simulink model "MovimientoTraslacionalSimulink2"  (R2023a)
settings: Solver=VariableStepAuto  StartTime=0.0  StopTime=10.0  RelTol=1e-3
values from neighbouring files (symbols this model uses):
  b1 = 1000    [MovTrasODE45.m]    (also in MovimientoTraslacionalSimulink.m)
  k1 = 16182    [MovTrasODE45.m]    (also in MovimientoTraslacionalSimulink.m)
  k2 = 19000    [MovTrasODE45.m]    (also in MovimientoTraslacionalSimulink.m)
  m1 = 290    [MovTrasODE45.m]    (also in MovimientoTraslacionalSimulink.m)
  m2 = 59    [MovTrasODE45.m]    (also in MovimientoTraslacionalSimulink.m)
settings Model: Creator=josel
settings OptimizationCC: ReuseModelBlockBuffer=off

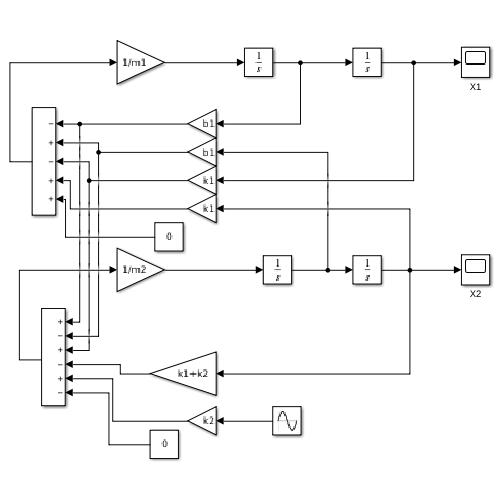
[thumbnail: Simulink's stored preview of the top-level diagram]
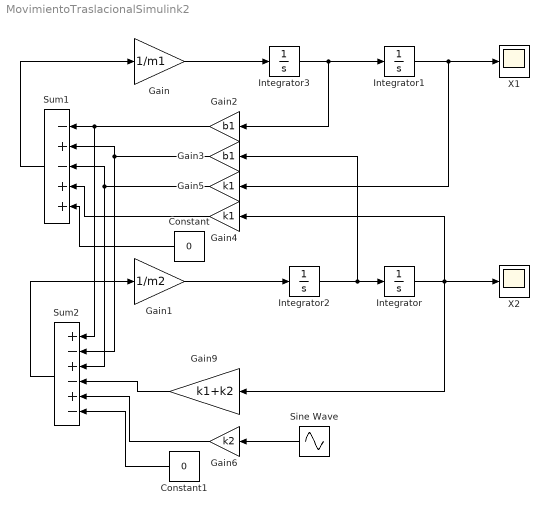
== system MovimientoTraslacionalSimulink2 ==
  Constant : Constant  Value=0
  Constant1 : Constant  Value=0
  Gain : Gain  Gain=1/m1
  Gain1 : Gain  Gain=1/m2
  Gain2 : Gain  Gain=b1
  Gain3 : Gain  Gain=b1
  Gain4 : Gain  Gain=k1
  Gain5 : Gain  Gain=k1
  Gain6 : Gain  Gain=k2
  Gain9 : Gain  Gain=k1+k2
  Integrator{,1..3} (4 alike) : Integrator
  Sine Wave : Sin  Amplitude=0.05  Frequency=0.5*pi  SampleTime=0
  Sum1 : Sum  Inputs=-+-++
  Sum2 : Sum  Inputs=+-+-+-
  X1 : Scope
  X2 : Scope
  wires:
  Gain/1 -> Integrator3/1
  Integrator3/1 -> Integrator1/1, Gain2/1
  Gain1/1 -> Integrator2/1
  Integrator2/1 -> Gain3/1, Integrator/1
  Integrator/1 -> X2/1, Gain4/1, Gain9/1
  Integrator1/1 -> Gain5/1, X1/1
  Sum1/1 -> Gain/1
  Gain2/1 -> Sum2/1, Sum1/1
  Gain3/1 -> Sum1/2, Sum2/2
  Gain5/1 -> Sum1/3, Sum2/3
  Gain4/1 -> Sum1/4
  Sum2/1 -> Gain1/1
  Sine Wave/1 -> Gain6/1
  Constant/1 -> Sum1/5
  Gain6/1 -> Sum2/5
  Constant1/1 -> Sum2/6
  Gain9/1 -> Sum2/4
